simulink model "ControlBorroso"  (R2015a)
settings: Solver=ode45  StartTime=0.0  StopTime=500.0  RelTol=1e-3
undefined symbols (not defined in the file): CBorr
libraries: fuzblock x1
settings Model: CovSFcnEnable=off  Creator=usuario_local  LastModifiedBy=Jota
settings SolverCC: ZeroCrossControl=DisableAll
settings DebuggingCC: SolverPrmCheckMsg=warning

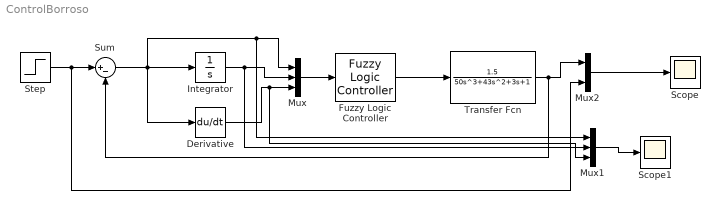
== system ControlBorroso ==
  Derivative : Derivative
  Fuzzy Logic Controller : fuzblock/Fuzzy Logic  Controller  fis=[CBorr]
  Integrator : Integrator
  Mux : Mux  Inputs=3
  Mux1 : Mux  Inputs=3
  Mux2 : Mux  Inputs=2
  Scope : Scope
  Scope1 : Scope
  Step : Step  SampleTime=0
  Sum : Sum  Inputs=|+-
  Transfer Fcn : TransferFcn  Numerator=[1.5]  Denominator=[50 43 3 1]
  wires:
  Step/1 -> Mux2/2, Sum/1
  Sum/1 -> Derivative/1, Integrator/1, Mux1/1, Mux/1
  Integrator/1 -> Mux1/2, Mux/2
  Fuzzy Logic Controller/1 -> Transfer Fcn/1
  Transfer Fcn/1 -> Sum/2, Mux2/1
  Mux2/1 -> Scope/1
  Derivative/1 -> Mux1/3, Mux/3
  Mux/1 -> Fuzzy Logic Controller/1
  Mux1/1 -> Scope1/1
